simulink model "aircraftSimulation"  (Simulink 8.4)
settings: Solver=ode3  StartTime=0.0  StopTime=10.0  FixedStep=sampleTime  RelTol=1e-3
settings Model: Creator=brtaylor  LastModifiedBy=brtaylor
settings DataIOCC: SignalLoggingSaveFormat=Dataset
settings OptimizationCC: ExpressionDepthLimit=128
settings DebuggingCC: UnderspecifiedInitializationDetection=Simplified  MergeDetectMultiDrivingBlocksExec=error  FcnCallInpInsideContextMsg=EnableAllAsError  StateNameClashWarn=none
settings GRTTargetCC: CombineOutputUpdateFcns=on  GRTInterface=off

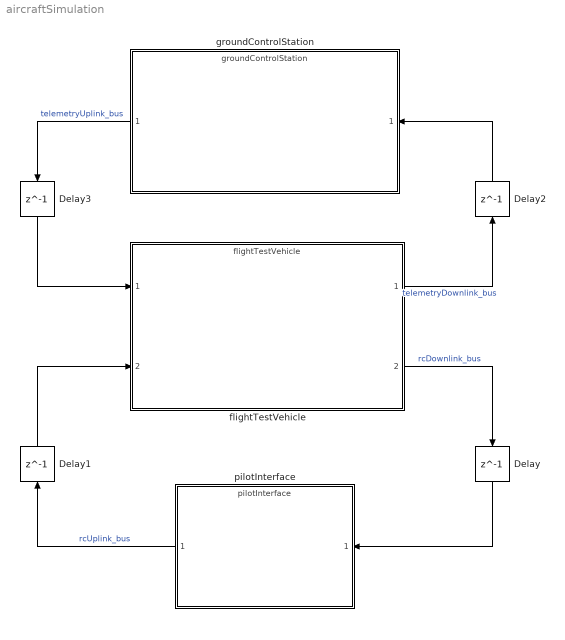
== system aircraftSimulation ==
  Delay{,1..3} (4 alike) : Delay  DelayLength=1
  flightTestVehicle : ModelReference  ModelNameDialog=flightTestVehicle.mdl  SimulationMode=Normal  ModelReferenceVersion=1.1  CopyOfModelName=flightTestVehicle.mdl  DefaultDataLogging=on
      mask Display: image(imread('vireo.jpg'))
  groundControlStation : ModelReference  ModelNameDialog=groundControlStation.mdl  SimulationMode=Normal  ModelReferenceVersion=1.1  CopyOfModelName=groundControlStation.mdl  DefaultDataLogging=on
      mask Display: image(imread('groundControlStation.jpg'))
  pilotInterface : ModelReference  ModelNameDialog=pilotInterface.mdl  SimulationMode=Normal  ModelReferenceVersion=1.1  CopyOfModelName=pilotInterface.mdl  DefaultDataLogging=on
      mask Display: image(imread('pilotInterface.png'))
  wires:
  flightTestVehicle/2 -> Delay/1  "rcDownlink_bus"
  pilotInterface/1 -> Delay1/1  "rcUplink_bus"
  groundControlStation/1 -> Delay3/1  "telemetryUplink_bus"
  flightTestVehicle/1 -> Delay2/1  "telemetryDownlink_bus"
  Delay/1 -> pilotInterface/1
  Delay1/1 -> flightTestVehicle/2
  Delay2/1 -> groundControlStation/1
  Delay3/1 -> flightTestVehicle/1
